simulink model "gm_untitled"  (R2021b)
settings: Solver=VariableStepAuto  StartTime=0.0  StopTime=0.001  RelTol=1e-3
libraries: simulink x1
settings Model: Creator=Green  LastModifiedBy=Green
settings OptimizationCC: BlockReduction=off  ConditionallyExecuteInputs=off
settings DebuggingCC: InheritedTsInSrcMsg=none

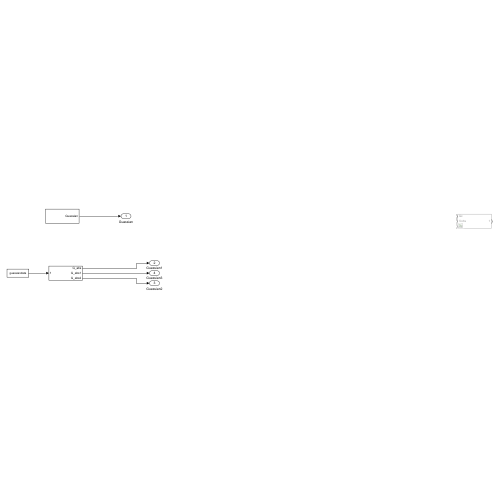
[thumbnail: Simulink's stored preview of the top-level diagram]
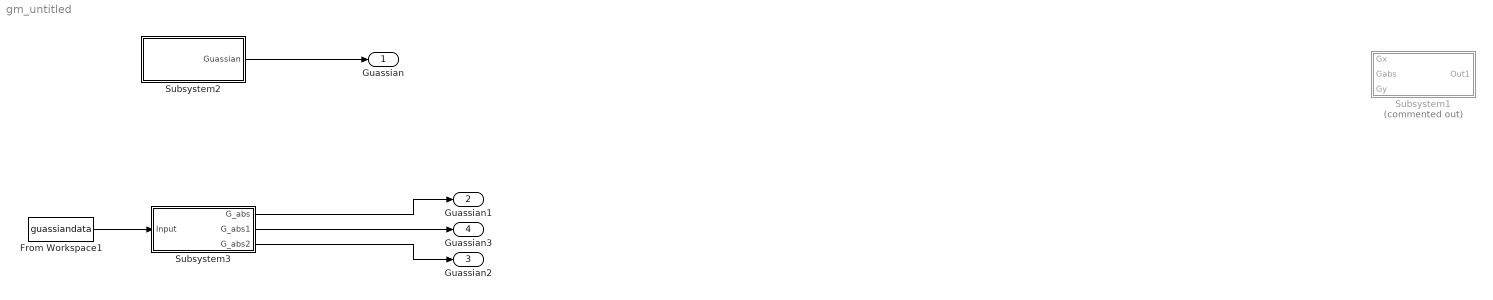
== system gm_untitled ==
  From Workspace1 : FromWorkspace  VariableName=guassiandata  SampleTime=-1  Interpolate=off  OutputAfterFinalValue=Holding final value
  Subsystem1 : Subsystem  Commented=on
  Subsystem2 : Subsystem
  Subsystem3 : Subsystem
  Guassian : Outport  VectorParamsAs1DForOutWhenUnconnected=off
  Guassian1 : Outport  Port=2  VectorParamsAs1DForOutWhenUnconnected=off
  Guassian2 : Outport  Port=3  VectorParamsAs1DForOutWhenUnconnected=off
  Guassian3 : Outport  Port=4  VectorParamsAs1DForOutWhenUnconnected=off
  wires:
  From Workspace1/1 -> Subsystem3/1(Input)
  Subsystem3/3(G_abs2) -> Guassian2/1
  Subsystem3/2(G_abs1) -> Guassian3/1
  Subsystem3/1(G_abs) -> Guassian1/1
  Subsystem2/1(Guassian) -> Guassian/1

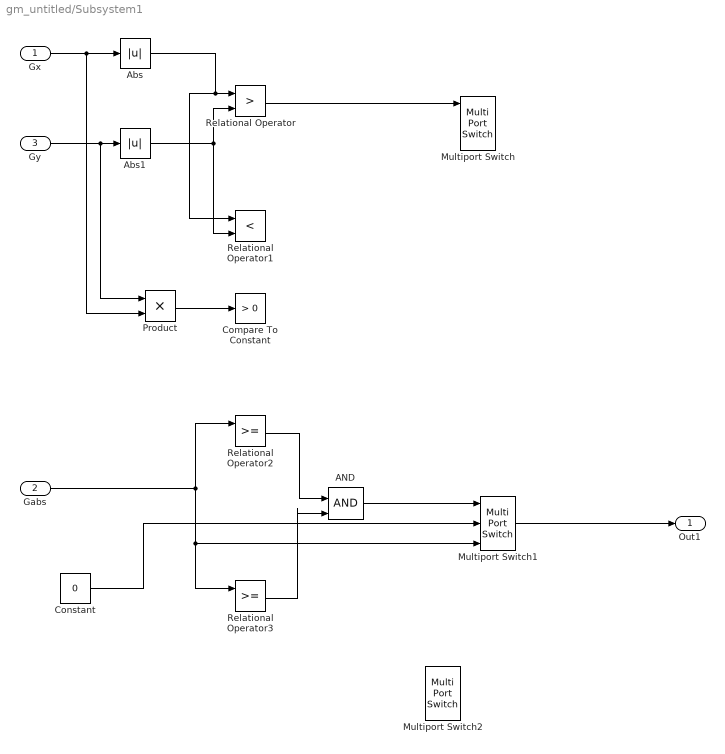
== system gm_untitled/Subsystem1 ==
  Gx : Inport
  Gabs : Inport  Port=2
  Gy : Inport  Port=3
  AND : Logic  IconShape=distinctive  AllPortsSameDT=off  OutDataTypeStr=boolean
  Abs : Abs
  Abs1 : Abs
  Compare To Constant : simulink/Logic and Bit Operations/Compare To Constant  relop=>  const=0  OutDataTypeStr=boolean
  Constant : Constant  Value=0
  Multiport Switch : MultiPortSwitch  DataPortOrder=Zero-based contiguous  Inputs=2  zeroidx=on
  Multiport Switch1 : MultiPortSwitch  DataPortOrder=Zero-based contiguous  Inputs=2  zeroidx=on
  Multiport Switch2 : MultiPortSwitch  DataPortOrder=Zero-based contiguous  Inputs=2  zeroidx=on
  Product : Product
  Relational Operator : RelationalOperator  Operator=>  OutDataTypeStr=boolean  RndMeth=Simplest
  Relational Operator1 : RelationalOperator  Operator=<  OutDataTypeStr=boolean  RndMeth=Simplest
  Relational Operator2 : RelationalOperator  OutDataTypeStr=boolean  RndMeth=Simplest
  Relational Operator3 : RelationalOperator  OutDataTypeStr=boolean  RndMeth=Simplest
  Out1 : Outport
  wires:
  Constant/1 -> Multiport Switch1/2
  Multiport Switch1/1 -> Out1/1
  AND/1 -> Multiport Switch1/1
  Relational Operator3/1 -> AND/2
  Relational Operator2/1 -> AND/1
  Gabs/1 -> Relational Operator2/1, Multiport Switch1/3, Relational Operator3/1
  Product/1 -> Compare To Constant/1
  Abs1/1 -> Relational Operator/2, Relational Operator1/2
  Abs/1 -> Relational Operator/1, Relational Operator1/1
  Gy/1 -> Abs1/1, Product/1
  Gx/1 -> Abs/1, Product/2
  Relational Operator/1 -> Multiport Switch/1

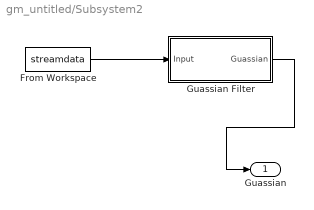
== system gm_untitled/Subsystem2 ==
  From Workspace : FromWorkspace  VariableName=streamdata  SampleTime=-1  Interpolate=off  OutputAfterFinalValue=Holding final value
  Guassian Filter : Subsystem
  Guassian : Outport
  wires:
  Guassian Filter/1(Guassian) -> Guassian/1
  From Workspace/1 -> Guassian Filter/1(Input)

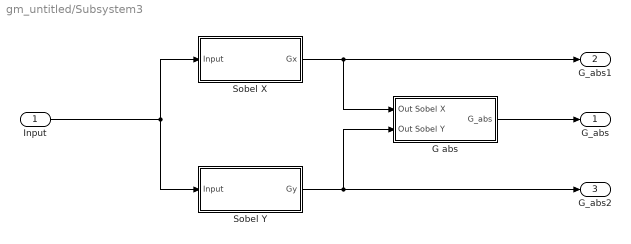
== system gm_untitled/Subsystem3 ==
  Input : Inport
  G abs : Subsystem
  Sobel X : Subsystem
  Sobel Y : Subsystem
  G_abs : Outport
  G_abs1 : Outport  Port=2
  G_abs2 : Outport  Port=3
  wires:
  G abs/1(G_abs) -> G_abs/1
  Sobel X/1(Gx) -> G abs/1(Out Sobel X), G_abs1/1
  Sobel Y/1(Gy) -> G abs/2(Out Sobel Y), G_abs2/1
  Input/1 -> Sobel X/1(Input), Sobel Y/1(Input)

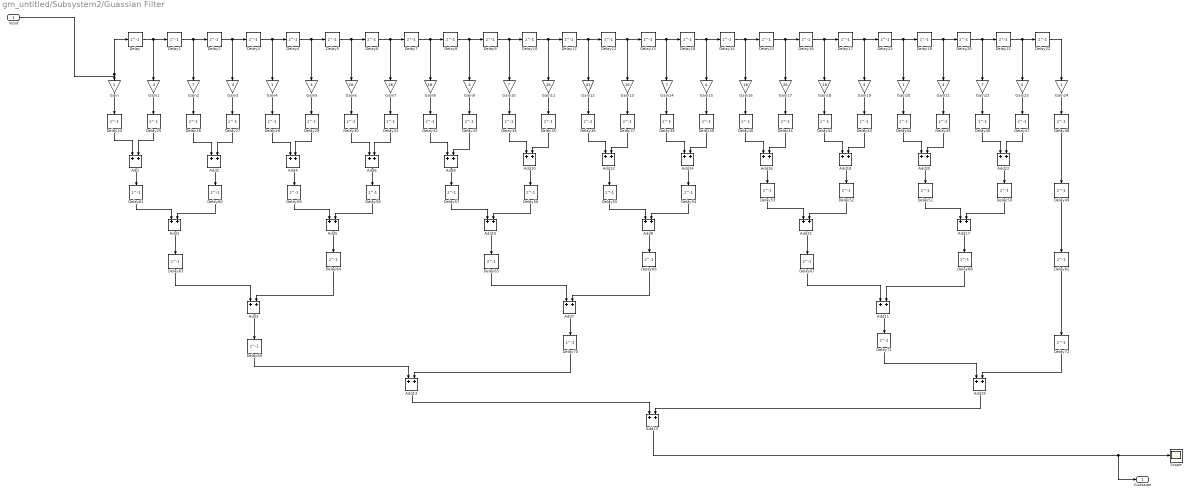
== system gm_untitled/Subsystem2/Guassian Filter ==
  Input : Inport
  Add{,1..23} (24 alike) : Sum
  Delay{,1..23,25..72} (72 alike) : Delay  DelayLength=1
  Delay24 : Delay  DelayLength=1  SampleTime=1e-8
  Gain{,4,20,24} (4 alike) : Gain  OutDataTypeStr=uint16
  Gain{1,3,5,9,15,19,21,23} (8 alike) : Gain  Gain=4  OutDataTypeStr=uint16
  Gain{2,10,14,22} (4 alike) : Gain  Gain=7  OutDataTypeStr=uint16
  Gain{7,11,13,17} (4 alike) : Gain  Gain=26  OutDataTypeStr=uint16
  Gain12 : Gain  Gain=41  OutDataTypeStr=uint16
  Gain{6,8,16,18} (4 alike) : Gain  Gain=16  OutDataTypeStr=uint16
  Scope : Scope
  Guassian : Outport  VectorParamsAs1DForOutWhenUnconnected=off
  wires:
  Delay27/1 -> Add2/2
  Input/1 -> Gain/1, Delay/1
  Gain/1 -> Delay24/1
  Delay6/1 -> Delay7/1, Gain7/1
  Delay33/1 -> Add8/2
  Delay8/1 -> Delay9/1, Gain9/1
  Add17/1 -> Delay68/1
  Delay19/1 -> Delay20/1, Gain21/1
  Delay43/1 -> Add18/2
  Delay54/1 -> Add9/2
  Add5/1 -> Delay64/1
  Add12/1 -> Delay55/1
  Delay57/1 -> Add15/1
  Delay25/1 -> Add/2
  Gain22/1 -> Delay46/1
  Add13/1 -> Add23/1
  Delay71/1 -> Add19/1
  Delay62/1 -> Delay72/1
  Gain3/1 -> Delay27/1
  Add/1 -> Delay61/1
  Add20/1 -> Delay51/1
  Delay7/1 -> Delay8/1, Gain8/1
  Gain23/1 -> Delay47/1
  Delay48/1 -> Delay49/1
  Delay18/1 -> Delay14/1, Gain15/1
  Delay49/1 -> Delay62/1
  Delay45/1 -> Add20/2
  Gain17/1 -> Delay41/1
  Gain21/1 -> Delay45/1
  Delay41/1 -> Add16/2
  Delay28/1 -> Add4/1
  Add23/1 -> Scope/1, Guassian/1
  Delay21/1 -> Gain23/1, Delay22/1
  Delay42/1 -> Add18/1
  Delay56/1 -> Add15/2
  Delay24/1 -> Add/1
  Gain24/1 -> Delay48/1
  Delay1/1 -> Gain2/1, Delay2/1
  Delay17/1 -> Delay23/1, Gain19/1
  Gain20/1 -> Delay44/1
  Delay40/1 -> Add16/1
  Delay65/1 -> Add7/1
  Gain2/1 -> Delay26/1
  Delay/1 -> Gain1/1, Delay1/1
  Delay29/1 -> Add4/2
  Delay34/1 -> Add10/1
  Gain9/1 -> Delay33/1
  Delay3/1 -> Gain4/1, Delay4/1
  Add8/1 -> Delay57/1
  Gain1/1 -> Delay25/1
  Add16/1 -> Delay53/1
  Delay20/1 -> Delay21/1, Gain22/1
  Gain8/1 -> Delay32/1
  Gain7/1 -> Delay31/1
  Gain6/1 -> Delay30/1
  Gain5/1 -> Delay29/1
  Delay30/1 -> Add6/1
  Delay46/1 -> Add22/1
  Add14/1 -> Delay54/1
  Add4/1 -> Delay59/1
  Gain15/1 -> Delay39/1
  Delay23/1 -> Delay19/1, Gain20/1
  Delay38/1 -> Add14/1
  Delay44/1 -> Add20/1
  Delay13/1 -> Delay18/1, Gain14/1
  Delay72/1 -> Add19/2
  Gain18/1 -> Delay42/1
  Gain16/1 -> Delay40/1
  Gain19/1 -> Delay43/1
  Delay4/1 -> Delay5/1, Gain5/1
  Add15/1 -> Delay65/1
  Gain4/1 -> Delay28/1
  Delay14/1 -> Delay15/1, Gain16/1
  Delay5/1 -> Delay6/1, Gain6/1
  Delay11/1 -> Delay12/1, Gain12/1
  Delay10/1 -> Delay11/1, Gain11/1
  Gain11/1 -> Delay35/1
  Gain10/1 -> Delay34/1
  Gain14/1 -> Delay38/1
  Gain12/1 -> Delay36/1
  Gain13/1 -> Delay37/1
  Delay15/1 -> Delay16/1, Gain17/1
  Delay32/1 -> Add8/1
  Delay36/1 -> Add12/1
  Delay37/1 -> Add12/2
  Delay12/1 -> Delay13/1, Gain13/1
  Delay16/1 -> Delay17/1, Gain18/1
  Delay9/1 -> Gain10/1, Delay10/1
  Add10/1 -> Delay56/1
  Delay22/1 -> Gain24/1
  Delay2/1 -> Gain3/1, Delay3/1
  Add2/1 -> Delay60/1
  Delay39/1 -> Add14/2
  Delay26/1 -> Add2/1
  Delay47/1 -> Add22/2
  Delay35/1 -> Add10/2
  Delay53/1 -> Add21/1
  Add19/1 -> Add23/2
  Add11/1 -> Delay71/1
  Delay69/1 -> Add13/1
  Delay61/1 -> Add1/1
  Add7/1 -> Delay70/1
  Add3/1 -> Delay69/1
  Add22/1 -> Delay50/1
  Delay60/1 -> Add1/2
  Delay31/1 -> Add6/2
  Delay58/1 -> Add5/2
  Delay59/1 -> Add5/1
  Add1/1 -> Delay63/1
  Delay64/1 -> Add3/2
  Delay70/1 -> Add13/2
  Delay55/1 -> Add9/1
  Add21/1 -> Delay67/1
  Add18/1 -> Delay52/1
  Delay63/1 -> Add3/1
  Delay66/1 -> Add7/2
  Delay51/1 -> Add17/1
  Add9/1 -> Delay66/1
  Delay68/1 -> Add11/2
  Delay67/1 -> Add11/1
  Delay52/1 -> Add21/2
  Add6/1 -> Delay58/1
  Delay50/1 -> Add17/2

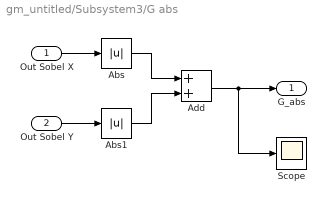
== system gm_untitled/Subsystem3/G abs ==
  Out Sobel X : Inport
  Out Sobel Y : Inport  Port=2
  Abs : Abs
  Abs1 : Abs
  Add : Sum
  Scope : Scope
  G_abs : Outport
  wires:
  Add/1 -> G_abs/1, Scope/1
  Abs1/1 -> Add/2
  Abs/1 -> Add/1
  Out Sobel Y/1 -> Abs1/1
  Out Sobel X/1 -> Abs/1

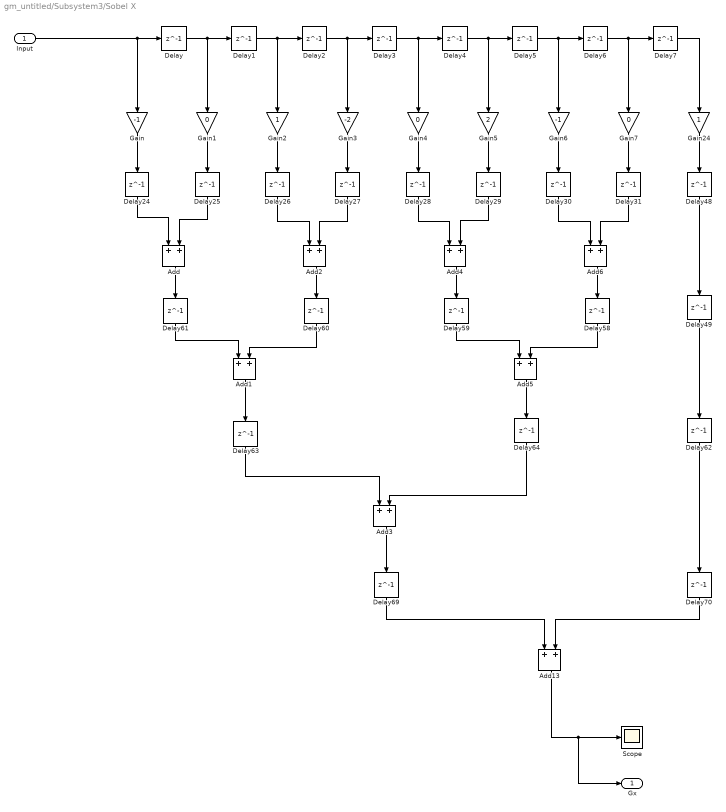
== system gm_untitled/Subsystem3/Sobel X ==
  Input : Inport
  Add{,1..6,13} (8 alike) : Sum
  Delay{,1..7,25..31,48..49,58..64,69..70} (26 alike) : Delay  DelayLength=1
  Delay24 : Delay  DelayLength=1  SampleTime=1e-8
  Gain : Gain  Gain=-1  ParamDataTypeStr=int16  OutDataTypeStr=int16
  Gain1 : Gain  Gain=0  OutDataTypeStr=int16
  Gain2 : Gain  OutDataTypeStr=int16
  Gain24 : Gain  ParamDataTypeStr=int16  OutDataTypeStr=int16
  Gain3 : Gain  Gain=-2  ParamDataTypeStr=int16  OutDataTypeStr=int16
  Gain4 : Gain  Gain=0  OutDataTypeStr=int16
  Gain5 : Gain  Gain=2  OutDataTypeStr=int16
  Gain6 : Gain  Gain=-1  ParamDataTypeStr=int16  OutDataTypeStr=int16
  Gain7 : Gain  Gain=0  OutDataTypeStr=int16
  Scope : Scope
  Gx : Outport  VectorParamsAs1DForOutWhenUnconnected=off
  wires:
  Delay62/1 -> Delay70/1
  Delay7/1 -> Gain24/1
  Add6/1 -> Delay58/1
  Delay69/1 -> Add13/1
  Add13/1 -> Scope/1, Gx/1
  Delay63/1 -> Add3/1
  Delay70/1 -> Add13/2
  Delay26/1 -> Add2/1
  Gain1/1 -> Delay25/1
  Delay58/1 -> Add5/2
  Delay59/1 -> Add5/1
  Delay29/1 -> Add4/2
  Delay60/1 -> Add1/2
  Delay64/1 -> Add3/2
  Delay31/1 -> Add6/2
  Delay28/1 -> Add4/1
  Add1/1 -> Delay63/1
  Delay61/1 -> Add1/1
  Add3/1 -> Delay69/1
  Add5/1 -> Delay64/1
  Input/1 -> Delay/1, Gain/1
  Delay27/1 -> Add2/2
  Delay6/1 -> Delay7/1, Gain7/1
  Delay2/1 -> Gain3/1, Delay3/1
  Gain/1 -> Delay24/1
  Add2/1 -> Delay60/1
  Gain4/1 -> Delay28/1
  Delay5/1 -> Delay6/1, Gain6/1
  Delay4/1 -> Delay5/1, Gain5/1
  Add4/1 -> Delay59/1
  Gain6/1 -> Delay30/1
  Gain7/1 -> Delay31/1
  Delay30/1 -> Add6/1
  Gain5/1 -> Delay29/1
  Delay3/1 -> Gain4/1, Delay4/1
  Gain2/1 -> Delay26/1
  Delay/1 -> Gain1/1, Delay1/1
  Delay24/1 -> Add/1
  Delay1/1 -> Gain2/1, Delay2/1
  Gain24/1 -> Delay48/1
  Delay49/1 -> Delay62/1
  Delay48/1 -> Delay49/1
  Add/1 -> Delay61/1
  Gain3/1 -> Delay27/1
  Delay25/1 -> Add/2

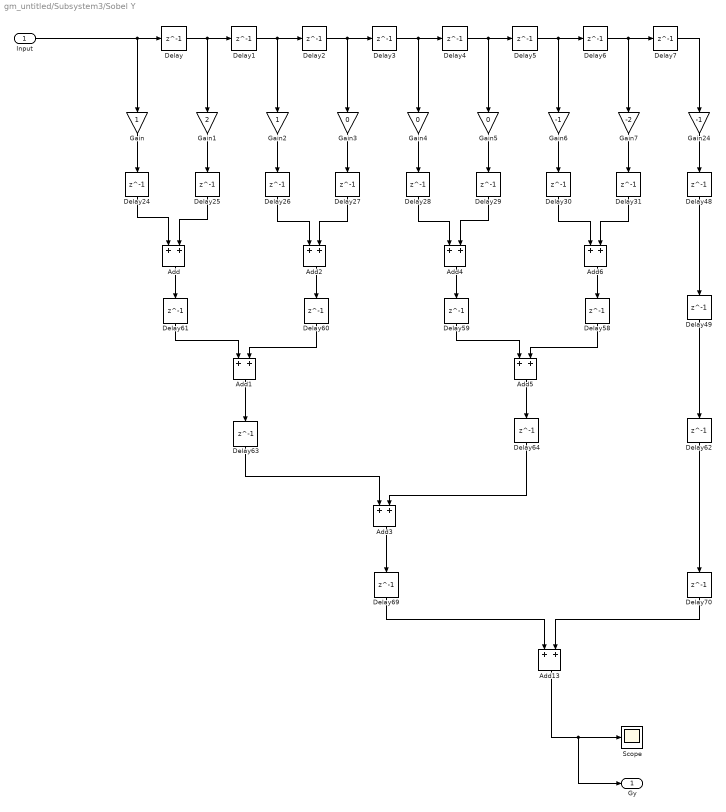
== system gm_untitled/Subsystem3/Sobel Y ==
  Input : Inport
  Add{,1..6,13} (8 alike) : Sum
  Delay{,1..7,25..31,48..49,58..64,69..70} (26 alike) : Delay  DelayLength=1
  Delay24 : Delay  DelayLength=1  SampleTime=1e-8
  Gain : Gain  OutDataTypeStr=int16
  Gain1 : Gain  Gain=2  OutDataTypeStr=int16
  Gain2 : Gain  OutDataTypeStr=int16
  Gain24 : Gain  Gain=-1  ParamDataTypeStr=int16  OutDataTypeStr=int16
  Gain3 : Gain  Gain=0  OutDataTypeStr=int16
  Gain4 : Gain  Gain=0  OutDataTypeStr=int16
  Gain5 : Gain  Gain=0  OutDataTypeStr=int16
  Gain6 : Gain  Gain=-1  ParamDataTypeStr=int16  OutDataTypeStr=int16
  Gain7 : Gain  Gain=-2  ParamDataTypeStr=int16  OutDataTypeStr=int16
  Scope : Scope
  Gy : Outport  VectorParamsAs1DForOutWhenUnconnected=off
  wires:
  Delay25/1 -> Add/2
  Gain3/1 -> Delay27/1
  Add/1 -> Delay61/1
  Delay48/1 -> Delay49/1
  Delay49/1 -> Delay62/1
  Gain24/1 -> Delay48/1
  Delay1/1 -> Delay2/1, Gain2/1
  Delay24/1 -> Add/1
  Delay/1 -> Delay1/1, Gain1/1
  Gain2/1 -> Delay26/1
  Delay3/1 -> Delay4/1, Gain4/1
  Gain5/1 -> Delay29/1
  Delay30/1 -> Add6/1
  Gain7/1 -> Delay31/1
  Gain6/1 -> Delay30/1
  Add4/1 -> Delay59/1
  Delay4/1 -> Gain5/1, Delay5/1
  Delay5/1 -> Gain6/1, Delay6/1
  Gain4/1 -> Delay28/1
  Add2/1 -> Delay60/1
  Gain/1 -> Delay24/1
  Delay2/1 -> Delay3/1, Gain3/1
  Delay6/1 -> Gain7/1, Delay7/1
  Delay27/1 -> Add2/2
  Input/1 -> Gain/1, Delay/1
  Add5/1 -> Delay64/1
  Add3/1 -> Delay69/1
  Delay61/1 -> Add1/1
  Add1/1 -> Delay63/1
  Delay28/1 -> Add4/1
  Delay31/1 -> Add6/2
  Delay64/1 -> Add3/2
  Delay60/1 -> Add1/2
  Delay29/1 -> Add4/2
  Delay59/1 -> Add5/1
  Delay58/1 -> Add5/2
  Gain1/1 -> Delay25/1
  Delay26/1 -> Add2/1
  Delay70/1 -> Add13/2
  Delay63/1 -> Add3/1
  Add13/1 -> Gy/1, Scope/1
  Delay69/1 -> Add13/1
  Add6/1 -> Delay58/1
  Delay7/1 -> Gain24/1
  Delay62/1 -> Delay70/1
